simulink subsystem "external_input_initializer"  (R2023a)
settings: Solver=VariableStepAuto  StartTime=0.0  StopTime=10.0  RelTol=1e-3
undefined symbols (not defined in the file): FLIGHT_MODE, flight_mode, joystick, Parameters, res, wait_time_s
libraries: vrlib x1
settings Model: Creator=thesa  LastModifiedBy=thesa

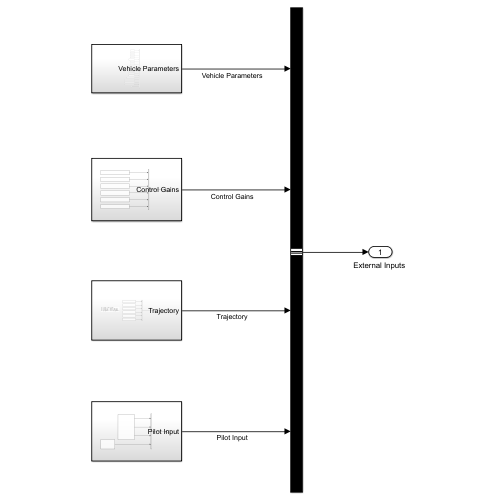
[thumbnail: Simulink's stored preview of the top-level diagram]
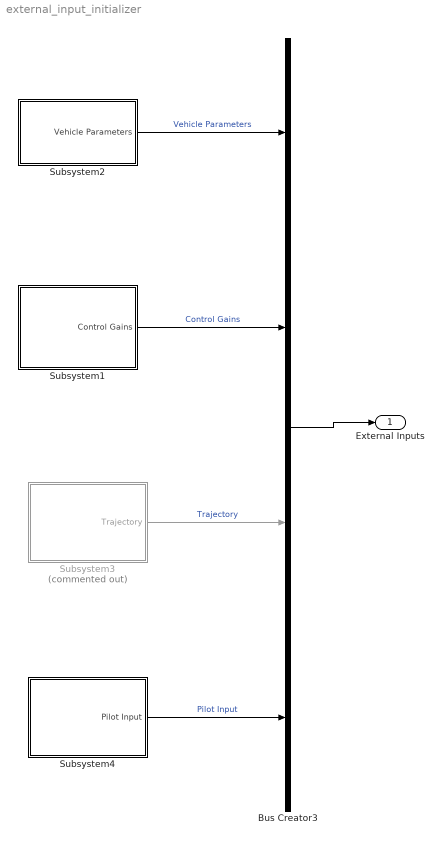
== system external_input_initializer ==
  Bus Creator3 : BusCreator  Inputs=4
  Subsystem1 : Subsystem
  Subsystem2 : Subsystem
  Subsystem3 : Subsystem  Commented=on
  Subsystem4 : Subsystem
  "External Inputs " : Outport
  wires:
  Subsystem4/1(Pilot Input) -> Bus Creator3/4  "Pilot Input"
  Subsystem2/1(Vehicle Parameters) -> Bus Creator3/1  "Vehicle Parameters"
  Subsystem3/1(Trajectory) -> Bus Creator3/3  "Trajectory"
  Bus Creator3/1 -> "External Inputs "/1
  Subsystem1/1(Control Gains) -> Bus Creator3/2  "Control Gains"

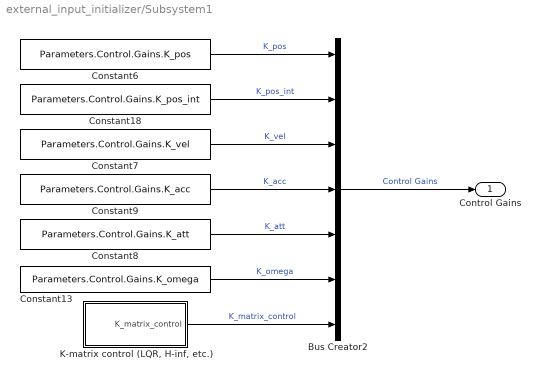
== system external_input_initializer/Subsystem1 ==
  " K-matrix control (LQR, H-inf, etc.)" : Subsystem
  Bus Creator2 : BusCreator  Inputs=7
  Constant13 : Constant  Value=Parameters.Control.Gains.K_omega
  Constant18 : Constant  Value=Parameters.Control.Gains.K_pos_int
  Constant6 : Constant  Value=Parameters.Control.Gains.K_pos
  Constant7 : Constant  Value=Parameters.Control.Gains.K_vel
  Constant8 : Constant  Value=Parameters.Control.Gains.K_att
  Constant9 : Constant  Value=Parameters.Control.Gains.K_acc
  Control Gains : Outport
  wires:
  " K-matrix control (LQR, H-inf, etc.)"/1(K_matrix_control) -> Bus Creator2/7  "K_matrix_control"
  Constant7/1 -> Bus Creator2/3  "K_vel"
  Constant6/1 -> Bus Creator2/1  "K_pos"
  Constant13/1 -> Bus Creator2/6  "K_omega"
  Bus Creator2/1 -> Control Gains/1  "Control Gains"
  Constant18/1 -> Bus Creator2/2  "K_pos_int"
  Constant9/1 -> Bus Creator2/4  "K_acc"
  Constant8/1 -> Bus Creator2/5  "K_att"

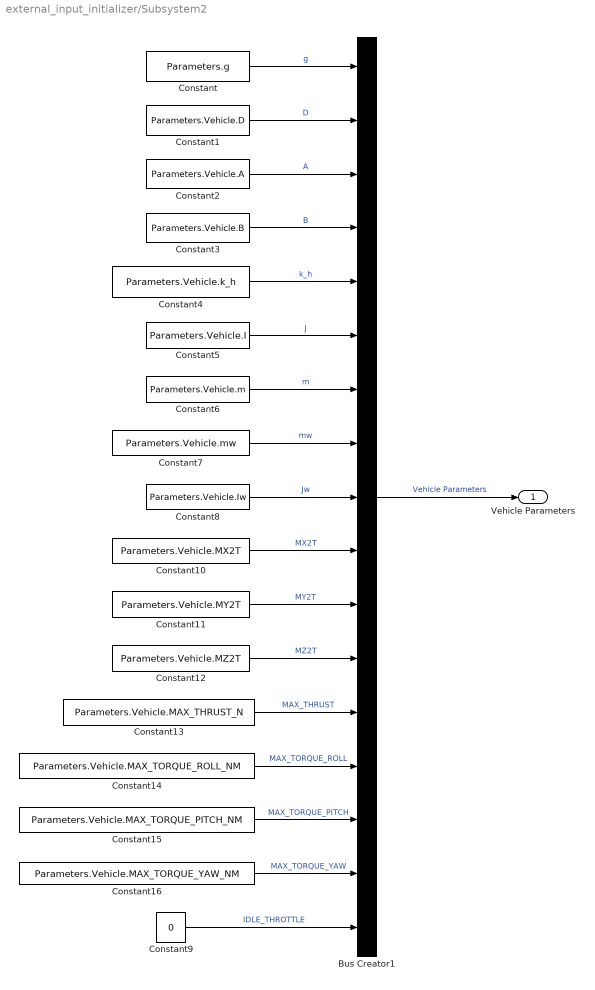
== system external_input_initializer/Subsystem2 ==
  Bus Creator1 : BusCreator  Inputs=17
  Constant : Constant  Value=Parameters.g
  Constant1 : Constant  Value=Parameters.Vehicle.D
  Constant10 : Constant  Value=Parameters.Vehicle.MX2T
  Constant11 : Constant  Value=Parameters.Vehicle.MY2T
  Constant12 : Constant  Value=Parameters.Vehicle.MZ2T
  Constant13 : Constant  Value=Parameters.Vehicle.MAX_THRUST_N
  Constant14 : Constant  Value=Parameters.Vehicle.MAX_TORQUE_ROLL_NM
  Constant15 : Constant  Value=Parameters.Vehicle.MAX_TORQUE_PITCH_NM
  Constant16 : Constant  Value=Parameters.Vehicle.MAX_TORQUE_YAW_NM
  Constant2 : Constant  Value=Parameters.Vehicle.A
  Constant3 : Constant  Value=Parameters.Vehicle.B
  Constant4 : Constant  Value=Parameters.Vehicle.k_h
  Constant5 : Constant  Value=Parameters.Vehicle.I
  Constant6 : Constant  Value=Parameters.Vehicle.m
  Constant7 : Constant  Value=Parameters.Vehicle.mw
  Constant8 : Constant  Value=Parameters.Vehicle.Iw
  Constant9 : Constant  Value=0
  Vehicle Parameters : Outport
  wires:
  Constant5/1 -> Bus Creator1/6  "J"
  Constant3/1 -> Bus Creator1/4  "B"
  Constant/1 -> Bus Creator1/1  "g"
  Constant1/1 -> Bus Creator1/2  "D"
  Constant2/1 -> Bus Creator1/3  "A"
  Constant4/1 -> Bus Creator1/5  "k_h"
  Bus Creator1/1 -> Vehicle Parameters/1  "Vehicle Parameters"
  Constant6/1 -> Bus Creator1/7  "m"
  Constant7/1 -> Bus Creator1/8  "mw"
  Constant8/1 -> Bus Creator1/9  "Jw"
  Constant10/1 -> Bus Creator1/10  "MX2T"
  Constant11/1 -> Bus Creator1/11  "MY2T"
  Constant12/1 -> Bus Creator1/12  "MZ2T"
  Constant13/1 -> Bus Creator1/13  "MAX_THRUST"
  Constant14/1 -> Bus Creator1/14  "MAX_TORQUE_ROLL"
  Constant15/1 -> Bus Creator1/15  "MAX_TORQUE_PITCH"
  Constant16/1 -> Bus Creator1/16  "MAX_TORQUE_YAW"
  Constant9/1 -> Bus Creator1/17  "IDLE_THROTTLE"

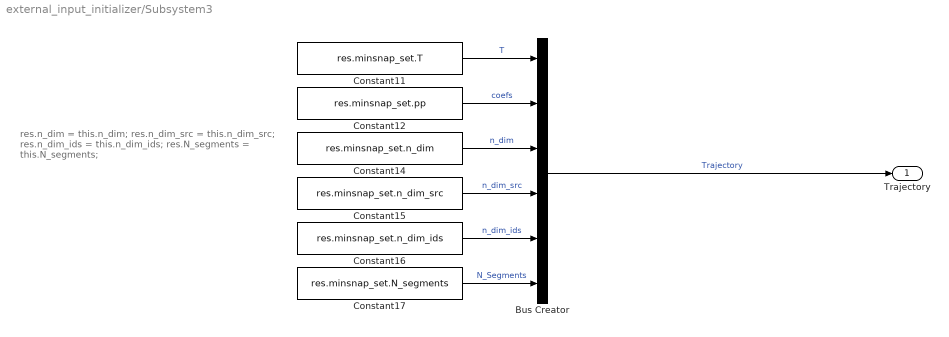
== system external_input_initializer/Subsystem3 ==
  note: res.n_dim = this.n_dim;
      | res.n_dim_src = this.n_dim_src;
      | res.n_dim_ids = this.n_dim_ids;
      | res.N_segments = this.N_segments;
  Bus Creator : BusCreator  Inputs=6
  Constant11 : Constant  Value=res.minsnap_set.T
  Constant12 : Constant  Value=res.minsnap_set.pp
  Constant14 : Constant  Value=res.minsnap_set.n_dim
  Constant15 : Constant  Value=res.minsnap_set.n_dim_src
  Constant16 : Constant  Value=res.minsnap_set.n_dim_ids
  Constant17 : Constant  Value=res.minsnap_set.N_segments
  Trajectory : Outport
  wires:
  Constant12/1 -> Bus Creator/2  "coefs"
  Constant14/1 -> Bus Creator/3  "n_dim"
  Constant11/1 -> Bus Creator/1  "T"
  Constant16/1 -> Bus Creator/5  "n_dim_ids"
  Bus Creator/1 -> Trajectory/1  "Trajectory"
  Constant15/1 -> Bus Creator/4  "n_dim_src"
  Constant17/1 -> Bus Creator/6  "N_Segments"

== system external_input_initializer/Subsystem4 ==
  Bus Creator4 : BusCreator  Inputs=4
  Subsystem : Subsystem
  Subsystem1 : Subsystem
  Pilot Input : Outport
  wires:
  Subsystem/1(sticks) -> Bus Creator4/1  "Sticks"
  Bus Creator4/1 -> Pilot Input/1  "Pilot Input"
  Subsystem1/1(Parameters) -> Bus Creator4/4  "Parameters"
  Subsystem/2(FLIGHT_MODE) -> Bus Creator4/2  "FLIGHT_MODE"
  Subsystem/3(ARMED) -> Bus Creator4/3  "ARMED"

== system external_input_initializer/Subsystem1/ K-matrix control (LQR, H-inf, etc.) ==
  Bus Creator : BusCreator  Inputs=4
  Constant1 : Constant  Value=Parameters.K_Control.K
  Constant2 : Constant  Value=Parameters.K_Control.EN
  Constant3 : Constant  Value=Parameters.K_Control.K_pos_int
  Subsystem : Subsystem
  K_matrix_control : Outport
  wires:
  Subsystem/1(ref) -> Bus Creator/4
  Constant3/1 -> Bus Creator/3  "K_pos_int"
  Constant2/1 -> Bus Creator/1  "EN"
  Constant1/1 -> Bus Creator/2  "K"
  Bus Creator/1 -> K_matrix_control/1  "K_matrix_control"

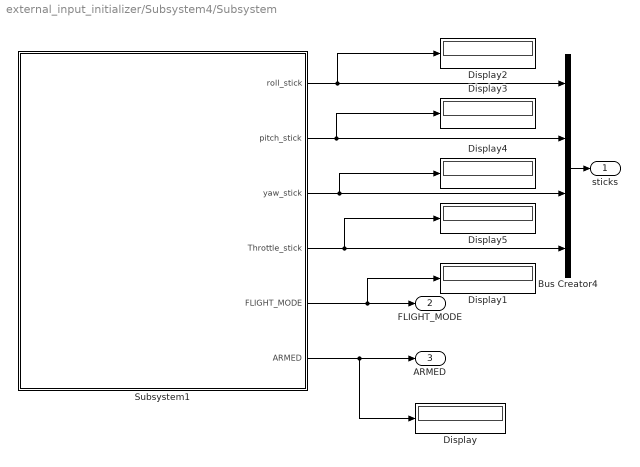
== system external_input_initializer/Subsystem4/Subsystem ==
  Bus Creator4 : BusCreator  Inputs=4
  Display{,1..5} (6 alike) : Display
  Subsystem1 : Subsystem  Variant=on  VariantControlMode=label  VariantControl=Choice  LabelModeActiveChoice=Choice_1
  sticks : Outport
  FLIGHT_MODE : Outport  Port=2
  ARMED : Outport  Port=3
  wires:
  Bus Creator4/1 -> sticks/1
  Subsystem1/1(roll_stick) -> Bus Creator4/1, Display2/1
  Subsystem1/2(pitch_stick) -> Bus Creator4/2, Display3/1
  Subsystem1/3(yaw_stick) -> Display4/1, Bus Creator4/3
  Subsystem1/4(Throttle_stick) -> Display5/1, Bus Creator4/4
  Subsystem1/5(FLIGHT_MODE) -> Display1/1, FLIGHT_MODE/1
  Subsystem1/6(ARMED) -> Display/1, ARMED/1

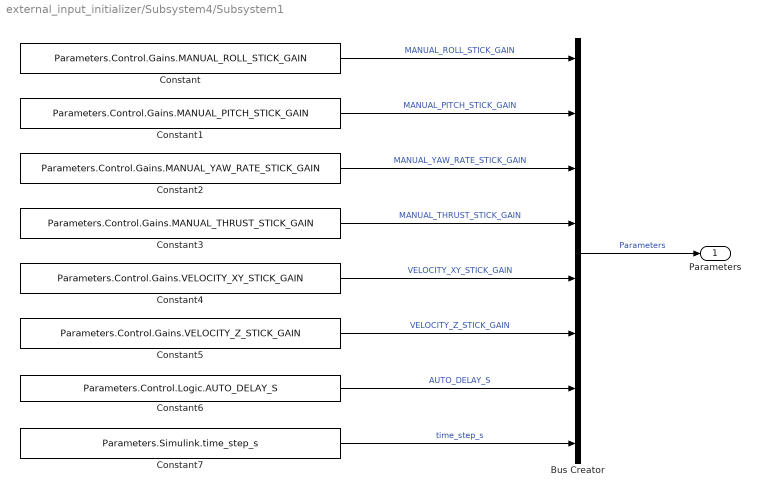
== system external_input_initializer/Subsystem4/Subsystem1 ==
  Bus Creator : BusCreator  Inputs=8
  Constant : Constant  Value=Parameters.Control.Gains.MANUAL_ROLL_STICK_GAIN
  Constant1 : Constant  Value=Parameters.Control.Gains.MANUAL_PITCH_STICK_GAIN
  Constant2 : Constant  Value=Parameters.Control.Gains.MANUAL_YAW_RATE_STICK_GAIN
  Constant3 : Constant  Value=Parameters.Control.Gains.MANUAL_THRUST_STICK_GAIN
  Constant4 : Constant  Value=Parameters.Control.Gains.VELOCITY_XY_STICK_GAIN
  Constant5 : Constant  Value=Parameters.Control.Gains.VELOCITY_Z_STICK_GAIN
  Constant6 : Constant  Value=Parameters.Control.Logic.AUTO_DELAY_S
  Constant7 : Constant  Value=Parameters.Simulink.time_step_s
  Parameters : Outport
  wires:
  Constant/1 -> Bus Creator/1  "MANUAL_ROLL_STICK_GAIN"
  Bus Creator/1 -> Parameters/1  "Parameters"
  Constant1/1 -> Bus Creator/2  "MANUAL_PITCH_STICK_GAIN"
  Constant2/1 -> Bus Creator/3  "MANUAL_YAW_RATE_STICK_GAIN"
  Constant3/1 -> Bus Creator/4  "MANUAL_THRUST_STICK_GAIN"
  Constant4/1 -> Bus Creator/5  "VELOCITY_XY_STICK_GAIN"
  Constant5/1 -> Bus Creator/6  "VELOCITY_Z_STICK_GAIN"
  Constant6/1 -> Bus Creator/7  "AUTO_DELAY_S"
  Constant7/1 -> Bus Creator/8  "time_step_s"

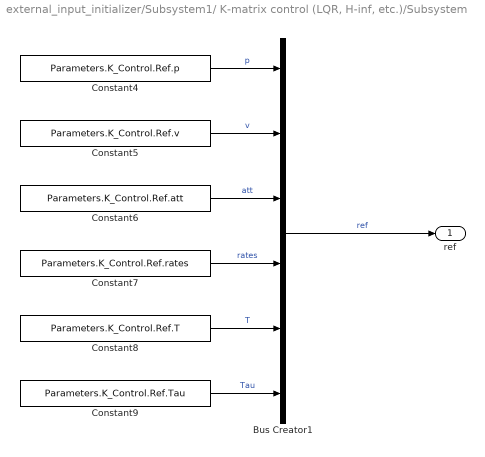
== system external_input_initializer/Subsystem1/ K-matrix control (LQR, H-inf, etc.)/Subsystem ==
  Bus Creator1 : BusCreator  Inputs=6
  Constant4 : Constant  Value=Parameters.K_Control.Ref.p
  Constant5 : Constant  Value=Parameters.K_Control.Ref.v
  Constant6 : Constant  Value=Parameters.K_Control.Ref.att
  Constant7 : Constant  Value=Parameters.K_Control.Ref.rates
  Constant8 : Constant  Value=Parameters.K_Control.Ref.T
  Constant9 : Constant  Value=Parameters.K_Control.Ref.Tau
  ref : Outport
  wires:
  Constant4/1 -> Bus Creator1/1  "p"
  Bus Creator1/1 -> ref/1  "ref"
  Constant6/1 -> Bus Creator1/3  "att"
  Constant7/1 -> Bus Creator1/4  "rates"
  Constant9/1 -> Bus Creator1/6  "Tau"
  Constant5/1 -> Bus Creator1/2  "v"
  Constant8/1 -> Bus Creator1/5  "T"

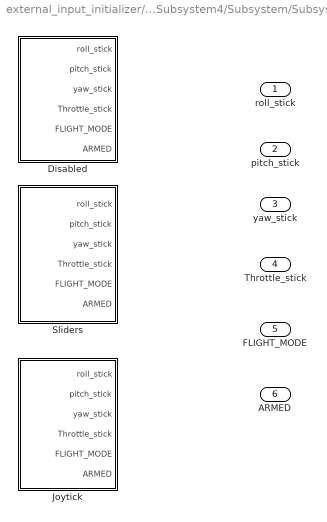
== system external_input_initializer/Subsystem4/Subsystem/Subsystem1 ==
  Disabled : Subsystem  VariantControl=Choice_1
  Joytick : Subsystem  VariantControl=Choice
  Sliders : Subsystem  VariantControl=Choice_2
  roll_stick : Outport
  pitch_stick : Outport  Port=2
  yaw_stick : Outport  Port=3
  Throttle_stick : Outport  Port=4
  FLIGHT_MODE : Outport  Port=5
  ARMED : Outport  Port=6

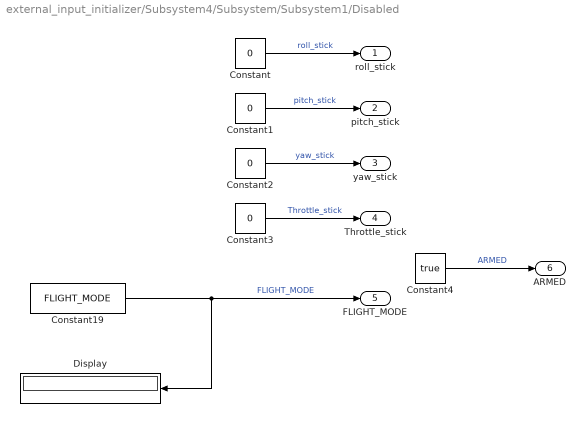
== system external_input_initializer/Subsystem4/Subsystem/Subsystem1/Disabled ==
  Constant{,1..3} (4 alike) : Constant  Value=0
  Constant19 : Constant  Value=FLIGHT_MODE
  Constant4 : Constant  Value=true
  Display : Display
  roll_stick : Outport
  pitch_stick : Outport  Port=2
  yaw_stick : Outport  Port=3
  Throttle_stick : Outport  Port=4
  FLIGHT_MODE : Outport  Port=5
  ARMED : Outport  Port=6
  wires:
  Constant3/1 -> Throttle_stick/1  "Throttle_stick"
  Constant1/1 -> pitch_stick/1  "pitch_stick"
  Constant/1 -> roll_stick/1  "roll_stick"
  Constant2/1 -> yaw_stick/1  "yaw_stick"
  Constant19/1 -> FLIGHT_MODE/1, Display/1  "FLIGHT_MODE"
  Constant4/1 -> ARMED/1  "ARMED"

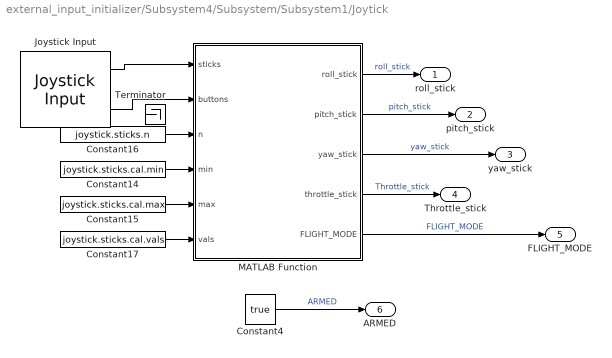
== system external_input_initializer/Subsystem4/Subsystem/Subsystem1/Joytick ==
  Constant14 : Constant  Value=joystick.sticks.cal.min
  Constant15 : Constant  Value=joystick.sticks.cal.max
  Constant16 : Constant  Value=joystick.sticks.n
  Constant17 : Constant  Value=joystick.sticks.cal.vals
  Constant4 : Constant  Value=true
  Joystick Input : vrlib/Joystick Input  joyid=1  adjustports=on  forcefeed=off
  MATLAB Function : MATLAB Function  TreatAsAtomicUnit=on
  Terminator : Terminator
  roll_stick : Outport
  pitch_stick : Outport  Port=2
  yaw_stick : Outport  Port=3
  Throttle_stick : Outport  Port=4
  FLIGHT_MODE : Outport  Port=5
  ARMED : Outport  Port=6
  wires:
  Constant15/1 -> MATLAB Function/5(max)
  Constant14/1 -> MATLAB Function/4(min)
  MATLAB Function/4(throttle_stick) -> Throttle_stick/1  "Throttle_stick"
  Constant16/1 -> MATLAB Function/3(n)
  Constant17/1 -> MATLAB Function/6(vals)
  Joystick Input/1 -> MATLAB Function/1(sticks)
  MATLAB Function/2(pitch_stick) -> pitch_stick/1  "pitch_stick"
  Joystick Input/2 -> MATLAB Function/2(buttons)
  ? -> Terminator/1
  MATLAB Function/1(roll_stick) -> roll_stick/1  "roll_stick"
  MATLAB Function/3(yaw_stick) -> yaw_stick/1  "yaw_stick"
  MATLAB Function/5(FLIGHT_MODE) -> FLIGHT_MODE/1  "FLIGHT_MODE"
  Constant4/1 -> ARMED/1  "ARMED"

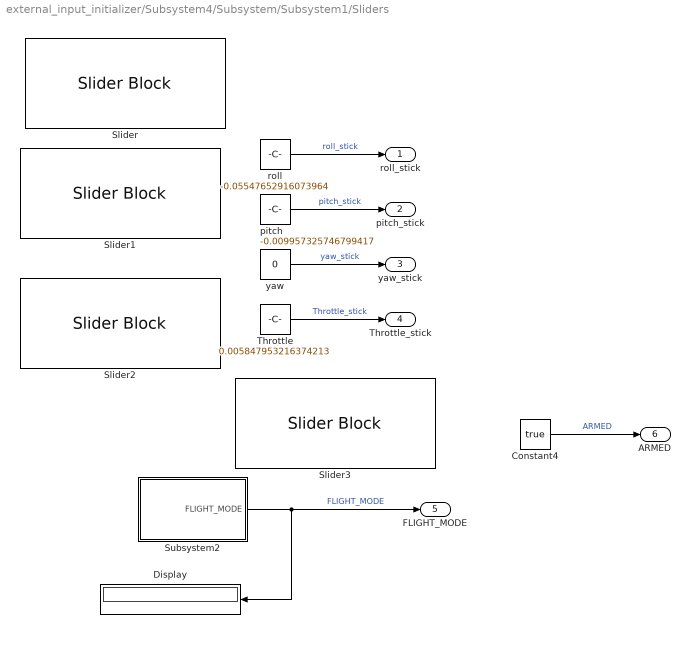
== system external_input_initializer/Subsystem4/Subsystem/Subsystem1/Sliders ==
  Constant4 : Constant  Value=true
  Display : Display
  Slider{,1..3} (4 alike) : SliderBlock  ScaleMin=-1  ScaleMax=1
  Subsystem2 : Subsystem
  Throttle : Constant  Value=0.005847953216374213
  pitch : Constant  Value=-0.009957325746799417
  roll : Constant  Value=-0.05547652916073964
  yaw : Constant  Value=0
  roll_stick : Outport
  pitch_stick : Outport  Port=2
  yaw_stick : Outport  Port=3
  Throttle_stick : Outport  Port=4
  FLIGHT_MODE : Outport  Port=5
  ARMED : Outport  Port=6
  wires:
  roll/1 -> roll_stick/1  "roll_stick"
  yaw/1 -> yaw_stick/1  "yaw_stick"
  pitch/1 -> pitch_stick/1  "pitch_stick"
  Throttle/1 -> Throttle_stick/1  "Throttle_stick"
  Subsystem2/1(FLIGHT_MODE) -> FLIGHT_MODE/1, Display/1  "FLIGHT_MODE"
  Constant4/1 -> ARMED/1  "ARMED"

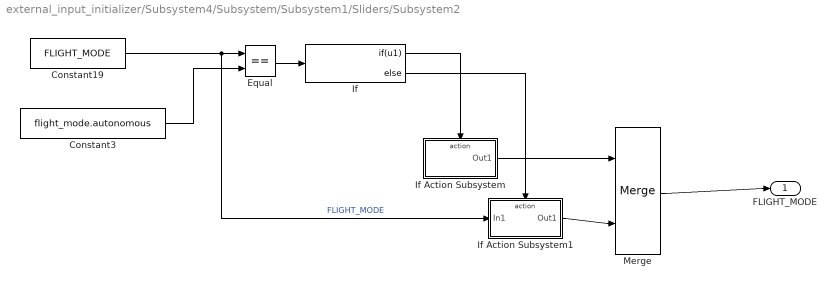
== system external_input_initializer/Subsystem4/Subsystem/Subsystem1/Sliders/Subsystem2 ==
  Constant19 : Constant  Value=FLIGHT_MODE
  Constant3 : Constant  Value=flight_mode.autonomous
  Equal : RelationalOperator  Operator===  OutDataTypeStr=boolean  RndMeth=Simplest  InputSameDT=off
  If : If  IfExpression=u1
  If Action Subsystem : Subsystem  TreatAsAtomicUnit=on
  If Action Subsystem1 : Subsystem  TreatAsAtomicUnit=on
  Merge : Merge
  FLIGHT_MODE : Outport
  wires:
  If/1 -> If Action Subsystem/Action
  If Action Subsystem1/1(Out1) -> Merge/2
  Merge/1 -> FLIGHT_MODE/1
  Constant19/1 -> If Action Subsystem1/1(In1), Equal/1  "FLIGHT_MODE"
  Constant3/1 -> Equal/2
  Equal/1 -> If/1
  If/2 -> If Action Subsystem1/Action
  If Action Subsystem/1(Out1) -> Merge/1

== system external_input_initializer/Subsystem4/Subsystem/Subsystem1/Sliders/Subsystem2/If Action Subsystem ==
  Action Port : ActionPort
  Clock : Clock
  Constant : Constant  Value=flight_mode.autonomous
  Constant1 : Constant  Value=flight_mode.position_hold
  Constant2 : Constant  Value=wait_time_s
  GreaterThan : RelationalOperator  Operator=<  OutDataTypeStr=boolean  RndMeth=Simplest  InputSameDT=off
  Multiport Switch1 : MultiPortSwitch  DataPortOrder=Zero-based contiguous  Inputs=2  DiagnosticForDefault=None  zeroidx=on  SaturateOnIntegerOverflow=off  InputSameDT=off
  Out1 : Outport
  wires:
  Constant2/1 -> GreaterThan/2
  Constant1/1 -> Multiport Switch1/3
  GreaterThan/1 -> Multiport Switch1/1
  Constant/1 -> Multiport Switch1/2
  Multiport Switch1/1 -> Out1/1
  Clock/1 -> GreaterThan/1

== system external_input_initializer/Subsystem4/Subsystem/Subsystem1/Sliders/Subsystem2/If Action Subsystem1 ==
  In1 : Inport
  Action Port : ActionPort
  Out1 : Outport
  wires:
  In1/1 -> Out1/1

== matlab function external_input_initializer/Subsystem4/Subsystem/Subsystem1/Joytick/MATLAB Function ==
  data: sticks input; roll_stick output; buttons input; n input; min input; max input; pitch_stick output; yaw_stick output; throttle_stick output; vals input; FLIGHT_MODE output
function [roll_stick, pitch_stick, yaw_stick, throttle_stick, FLIGHT_MODE] = fcn(sticks, buttons, n, min, max, vals)
joystick.sticks.raw = sticks;
joystick.buttons.raw = buttons;
joystick.sticks.n = n;
joystick.sticks.cal.min = min;
joystick.sticks.cal.max = max;
joystick.sticks.cal.vals = vals;

ROLL_STICK = 1;
PITCH_STICK = 2;
THROTTLE_STICK = 3;
YAW_STICK = 5;
AUX1_STICK = 4;

StickMap = [...
    ROLL_STICK
    PITCH_STICK
    YAW_STICK
    THROTTLE_STICK
    AUX1_STICK];

ROLL_STICK_POL = 1;
PITCH_STICK_POL = -1;
THROTTLE_STICK_POL = -1;
YAW_STICK_POL = 1;
AUX1_STICK_POL = 1;

StickPol = [...
    ROLL_STICK_POL
    PITCH_STICK_POL
    YAW_STICK_POL
    THROTTLE_STICK_POL
    AUX1_STICK_POL];

% tol = 1E-12;
deadzone_RPY = 0.05; %sticks are not perfectly centered 
deadzone_Z = 0.05;
joystick = lib.joystick.apply_cal(joystick);
mapped_sticks = joystick.sticks.cal.vals(StickMap);
mapped_sticks = mapped_sticks(:).*StickPol(:);
roll_stick = lib.math.apply_deadzone(mapped_sticks(1),deadzone_RPY,0);
pitch_stick = lib.math.apply_deadzone(mapped_sticks(2),deadzone_RPY,0);
yaw_stick = lib.math.apply_deadzone(mapped_sticks(3),deadzone_RPY,0);
throttle_stick = lib.math.apply_deadzone(mapped_sticks(4),deadzone_Z,0);

button_case = 0;
flight_mode_buttons = buttons(4:5);
if flight_mode_buttons(1) == 0 && flight_mode_buttons(2) == 0
    button_case = 0;
elseif flight_mode_buttons(1) == 1
    button_case = 1;
elseif flight_mode_buttons(2) == 1
    button_case = 2;
end


switch button_case
    case 2
        FLIGHT_MODE = flight_mode.autonomous;
    case 1
        FLIGHT_MODE = flight_mode.attitude_control;
        % FLIGHT_MODE = flight_mode.position_control;
    case 0
        % FLIGHT_MODE = flight_mode.attitude_control;
        FLIGHT_MODE = flight_mode.position_control;
    otherwise 
        FLIGHT_MODE = flight_mode.position_hold;
end

end
